simulink model "ampel_steuerung"  (R2024b)
settings: Solver=VariableStepAuto  StartTime=0.0  StopTime=inf  RelTol=1e-3
settings Model: Creator=Steve Kinfack  LastModifiedBy=Steve Kinfack

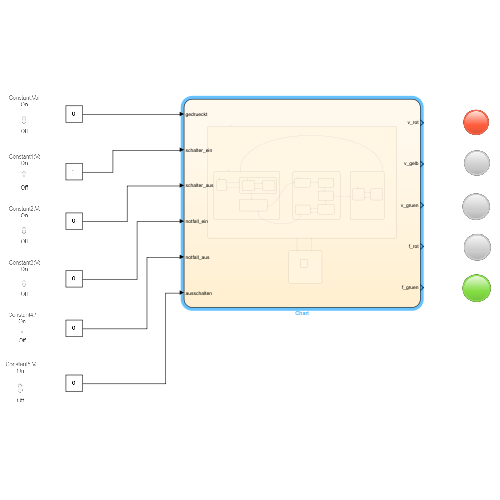
[thumbnail: Simulink's stored preview of the top-level diagram]
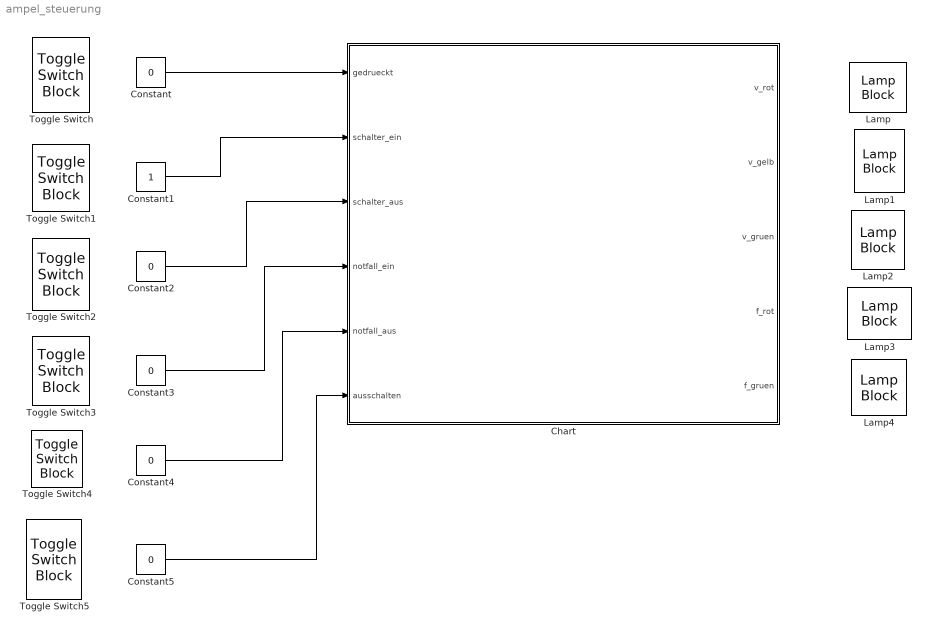
== system ampel_steuerung ==
  Chart : Stateflow chart  TreatAsAtomicUnit=on
  Constant{,2..5} (5 alike) : Constant  Value=0
  Constant1 : Constant
  Lamp{,1..4} (5 alike) : LampBlock  LabelPosition=Hide
  Toggle Switch{,1..5} (6 alike) : ToggleSwitchBlock
      settings: Values={{'Off', 'On'}, [0 1]}
  wires:
  Constant2/1 -> Chart/3(schalter_aus)
  Constant1/1 -> Chart/2(schalter_ein)
  Constant/1 -> Chart/1(gedrueckt)
  Constant3/1 -> Chart/4(notfall_ein)
  Constant4/1 -> Chart/5(notfall_aus)
  Constant5/1 -> Chart/6(ausschalten)

== stateflow chart ampel_steuerung/Chart ==
  state Normaler_betrieb
    state Startvorgang
      state A
        state Gelb_blink_und_f_rot
          entry:
          v_gelb = 0;
          f_rot = 0;
          exit:
          v_gelb = 1;
        state Gelb_blink_und_f_rot1
          entry:
          v_gelb = 1;
          f_rot = 0;
          exit:
          v_gelb = 0;
        (default) -> Gelb_blink_und_f_rot
        Gelb_blink_und_f_rot -> Gelb_blink_und_f_rot1 : after(1, sec)
        Gelb_blink_und_f_rot1 -> Gelb_blink_und_f_rot : after(1, sec)
      state Ampel_Aus
        entry:
        v_rot = 1;
        v_gelb = 1;
        v_gruen = 1;
        f_rot = 1;
        f_gruen = 1;
      state Verkehr_wechsel_von_gelb_auf_rot
        entry:
        v_gelb = 1;
        v_rot = 0;
      (default) -> Ampel_Aus
      Ampel_Aus -> A : [schalter_ein]
      A -> Ampel_Aus [order 1] : [schalter_aus]
      A -> Verkehr_wechsel_von_gelb_auf_rot [order 2] : after(10, sec)
    state Betrieb
      state F_wechselt_von_gruen_auf_rot
        entry:
        f_gruen = 1;
        f_rot = 0;
      state F_wechselt_von_rot_auf_gruen
        entry:
        f_rot = 1;
        f_gruen = 0;
        exit:
        f_gruen = 1;
      state V_schaltet_von_rot_auf_rot_gelb
        entry:
        v_rot = 0;
        v_gelb = 0;
        exit:
        v_rot = 1;
        v_gelb = 1
      state V_schaltet_von_rot_gelb_auf_gruen
        entry:
        v_rot = 1;
        v_gelb = 1;
        v_gruen = 0;
        exit:
        v_gruen = 1;
      state V_schaltet_von_gruen_auf_gelb
        entry:
        v_gruen = 1;
        v_gelb = 0;
        exit:
        v_gelb = 1;
      (default) -> F_wechselt_von_rot_auf_gruen
      F_wechselt_von_rot_auf_gruen -> F_wechselt_von_gruen_auf_rot : after(15, sec)
      F_wechselt_von_gruen_auf_rot -> V_schaltet_von_rot_auf_rot_gelb : after(2, sec)
      V_schaltet_von_rot_auf_rot_gelb -> V_schaltet_von_rot_gelb_auf_gruen [order 1] : after(2, sec)
      V_schaltet_von_rot_gelb_auf_gruen -> V_schaltet_von_gruen_auf_gelb [order 1] : after(40, sec)
      V_schaltet_von_rot_gelb_auf_gruen -> V_schaltet_von_gruen_auf_gelb [order 2] : after(15, sec)[gedrueckt]
    state Ausschalt_vorgang
      state V_blink_gelb
        entry:
        v_gelb = 0;
        exit:
        v_gelb = 1;
      state V_blink_gelb1
        entry:
        v_gelb = 1;
        exit:
        v_gelb = 0;
      (default) -> V_blink_gelb
      V_blink_gelb -> V_blink_gelb1 : after(1, sec)
      V_blink_gelb1 -> V_blink_gelb : after(1, sec)
    Ausschalt_vorgang -> Startvorgang : after(10, sec)
    (default) -> Startvorgang
    Verkehr_wechsel_von_gelb_auf_rot -> F_wechselt_von_rot_auf_gruen : after(5, sec)
    V_schaltet_von_rot_auf_rot_gelb -> Ausschalt_vorgang [order 2] : [ausschalten]
    V_schaltet_von_gruen_auf_gelb -> Verkehr_wechsel_von_gelb_auf_rot : after(2, sec)
  state Notfall
    state emergency
      entry:
      v_rot = 0;
      v_gelb = 1;
      v_gruen = 1;
      f_rot = 0;
      f_gruen = 1;
  (default) -> Normaler_betrieb
  Normaler_betrieb -> Notfall : [notfall_ein]
  Notfall -> Normaler_betrieb : [notfall_aus]
  data: v_rot output =1; v_gelb output =1; v_gruen output =1; f_rot output =1; f_gruen output =1; gedrueckt input; schalter_ein input; schalter_aus input; notfall_ein input; notfall_aus input; ausschalten input
